simulink model "B2_comparison_tool"  (R2021b)
settings: Solver=VariableStepAuto  StartTime=0.0  StopTime=10  RelTol=1e-3
values from neighbouring files (symbols this model uses):
  K_act = 50    [A10_simple_plant.m]    (also in A11_setup_script_pprz.m = 20; A1_setup_script.m = 20)
  K_act_inner = K_act*eye(4)    [A11_setup_script_pprz.m]    (also in A1_setup_script.m)
  K_ec_u = 1.5    [A11_setup_script_pprz.m]    (also in A1_setup_script.m = 5)
  K_ec_v = 1.5    [A11_setup_script_pprz.m]    (also in A1_setup_script.m = 5)
  K_ec_w = 1.5    [A11_setup_script_pprz.m]    (also in A1_setup_script.m = 5)
  K_u_d = 2.5    [A11_setup_script_pprz.m]    (also in A1_setup_script.m = 7)
  K_v_d = 2.5    [A11_setup_script_pprz.m]    (also in A1_setup_script.m = 7)
  K_w_d = 2.5    [A11_setup_script_pprz.m]    (also in A1_setup_script.m = 7)
  max_motor_rate = 30000    [A11_setup_script_pprz.m]    (also in A1_setup_script.m)
  max_omega_motor = 11000    [A11_setup_script_pprz.m]    (also in A1_setup_script.m)
  omega_c_motors = 50    [A11_setup_script_pprz.m]    (also in A1_setup_script.m)
  sampling_time = 1/frequency    (= 0.002)    [A11_setup_script_pprz.m]    (also in A12_sim_multi_run.m; A1_setup_script.m; A6_slow_actuator.m)
undefined symbols (not defined in the file or in its folder): K_ec_d_p, K_ec_d_q, K_ec_d_r, K_ec_dd_p, K_ec_dd_q, K_ec_dd_r, K_ec_p, K_ec_q, K_ec_r, K_p, K_p_d, K_p_dd, K_q, K_q_d, K_q_dd, K_r, K_r_d, K_r_dd
libraries: dspinverses x16, simulink_extras x8, aerolibutil x2, sharedutil x2, aerolibbdyn x2, aerolibatmos2 x2
(part 4 of 5)

== system B2_comparison_tool/System 1 - Old/INDI w// RSPI/ERROR CONTROLLER VELOCITY ==
  u_ref : Inport
  v_ref : Inport  Port=2
  w_ref : Inport  Port=3
  Gain : Gain  Gain=10
  Gain2 : Gain  Gain=10
  Gain4 : Gain  Gain=10
  Sum : Sum  Inputs=|+-
  Sum3 : Sum  Inputs=|+-
  Sum6 : Sum  Inputs=|+-
  ud_ec : Outport
  vd_ec : Outport  Port=2
  wd_ec : Outport  Port=3
  wires:
  u_ref/1 -> Sum/1
  Sum/1 -> Gain/1
  Gain/1 -> ud_ec/1
  Sum3/1 -> Gain2/1
  v_ref/1 -> Sum3/1
  Gain2/1 -> vd_ec/1
  Sum6/1 -> Gain4/1
  w_ref/1 -> Sum6/1
  [Vx_earth] -> Sum/2
  [Vz_earth] -> Sum6/2
  [Vy_earth] -> Sum3/2
  Gain4/1 -> wd_ec/1

== system B2_comparison_tool/System 1 - Old/INDI w// RSPI/INTERNAL REFERENCE MODEL ATTITUDE ==
  phi_cmd : Inport
  theta_cmd : Inport  Port=2
  psi_cmd : Inport  Port=3
  Gain1 : Gain  Gain=10
  Gain10 : Gain  Gain=20
  Gain11 : Gain  Gain=20
  Gain7 : Gain  Gain=5
  Gain8 : Gain  Gain=20
  Gain9 : Gain  Gain=5
  Integrator{,1..5} (6 alike) : Integrator
  Subsystem : Subsystem
  Subsystem1 : Subsystem
  Sum{1,11,16,20..22} (6 alike) : Sum  Inputs=|+-
  pd_ref : Outport
  qd_ref : Outport  Port=2
  rd_ref : Outport  Port=3
  p_ref : Outport  Port=4
  q_ref : Outport  Port=5
  r_ref : Outport  Port=6
  phi_ref : Outport  Port=7
  theta_ref : Outport  Port=8
  psi_ref : Outport  Port=9
  wires:
  Integrator1/1 -> Sum11/2, theta_ref/1
  Integrator2/1 -> p_ref/1, Subsystem1/1(p), Sum21/2
  Gain11/1 -> rd_ref/1, Integrator4/1
  Subsystem1/1(dphi) -> Integrator3/1
  Subsystem1/3(dpsi) -> Integrator5/1
  Subsystem1/2(dtheta) -> Integrator1/1
  Subsystem/2(q) -> Sum16/1
  Subsystem/1(p) -> Sum21/1
  Gain9/1 -> Subsystem/1(dphi)
  Subsystem/3(r) -> Sum22/1
  Gain8/1 -> qd_ref/1, Integrator/1
  Sum21/1 -> Gain10/1
  Gain7/1 -> Subsystem/2(dtheta)
  Sum11/1 -> Gain7/1
  Sum22/1 -> Gain11/1
  Sum16/1 -> Gain8/1
  Integrator3/1 -> phi_ref/1, Sum20/2
  Sum20/1 -> Gain9/1
  Integrator4/1 -> r_ref/1, Subsystem1/3(r), Sum22/2
  Gain10/1 -> pd_ref/1, Integrator2/1
  Integrator/1 -> q_ref/1, Subsystem1/2(q), Sum16/2
  phi_cmd/1 -> Sum20/1
  theta_cmd/1 -> Sum11/1
  psi_cmd/1 -> Sum1/1
  Integrator5/1 -> Sum1/2, psi_ref/1
  Gain1/1 -> Subsystem/3(dpsi)
  Sum1/1 -> Gain1/1

== system B2_comparison_tool/System 1 - Old/INDI w// RSPI/INTERNAL REFERENCE MODEL VELOCITY ==
  u_cmd : Inport
  v_cmd : Inport  Port=2
  w_cmd : Inport  Port=3
  Gain1 : Gain  Gain=2
  Gain7 : Gain  Gain=2
  Gain9 : Gain  Gain=2
  Integrator1 : Integrator
  Integrator3 : Integrator
  Integrator5 : Integrator
  Sum1 : Sum  Inputs=|+-
  Sum11 : Sum  Inputs=|+-
  Sum20 : Sum  Inputs=|+-
  ud_ref : Outport
  vd_ref : Outport  Port=2
  wd_ref : Outport  Port=3
  u_ref : Outport  Port=4
  v_ref : Outport  Port=5
  w_ref : Outport  Port=6
  wires:
  Integrator1/1 -> w_ref/1, Sum11/2
  Gain7/1 -> Integrator1/1, wd_ref/1
  Gain9/1 -> ud_ref/1, Integrator3/1
  v_cmd/1 -> Sum1/1
  Sum11/1 -> Gain7/1
  Integrator3/1 -> Sum20/2, u_ref/1
  Sum20/1 -> Gain9/1
  u_cmd/1 -> Sum20/1
  w_cmd/1 -> Sum11/1
  Integrator5/1 -> Sum1/2, v_ref/1
  Gain1/1 -> vd_ref/1, Integrator5/1
  Sum1/1 -> Gain1/1

== system B2_comparison_tool/System 0 - New/Equations of Motion/Vehicle Dynamics/Disturbance Block ==
  Step : Step  Time=2  After=60  SampleTime=0
  Sum : Sum  Inputs=|++
  Total Disturbance : Outport
  wires:
  Step/1 -> Sum/1
  Sum/1 -> Total Disturbance/1

== system B2_comparison_tool/System 0 - New/Equations of Motion/Vehicle Dynamics/Omega_I_Omega ==
  pqr_body : Inport
  Inertia : Inport  Port=2
  3x3 Cross Product : sharedutil/3x3 Cross Product  aMode=aMode
      settings: SourceProductBaseCode=AE,PW,DR,MT,UV,VE
  Matrix Multiply1 : Product  Multiplication=Matrix(*)
  Final product : Outport
  wires:
  Inertia/1 -> Matrix Multiply1/1
  Matrix Multiply1/1 -> 3x3 Cross Product/2
  3x3 Cross Product/1 -> Final product/1
  pqr_body/1 -> 3x3 Cross Product/1, Matrix Multiply1/2

== system B2_comparison_tool/System 0 - New/INDI Cascaded/INTERNAL REFERENCE MODEL ATTITUDE/Subsystem ==
  dphi : Inport
  dtheta : Inport  Port=2
  dpsi : Inport  Port=3
  Demux4 : Demux  Outputs=3
  Matrix Multiply2 : Product  Multiplication=Matrix(*)
  Vector Concatenate1 : Concatenate  NumInputs=3
  p : Outport
  q : Outport  Port=2
  r : Outport  Port=3
  wires:
  Vector Concatenate1/1 -> Matrix Multiply2/2
  [R] -> Matrix Multiply2/1
  dphi/1 -> Vector Concatenate1/1
  dtheta/1 -> Vector Concatenate1/2
  Matrix Multiply2/1 -> Demux4/1
  dpsi/1 -> Vector Concatenate1/3
  Demux4/3 -> r/1
  Demux4/1 -> p/1
  Demux4/2 -> q/1

== system B2_comparison_tool/System 0 - New/INDI Cascaded/INTERNAL REFERENCE MODEL ATTITUDE/Subsystem1 ==
  p : Inport
  q : Inport  Port=2
  r : Inport  Port=3
  Demux4 : Demux  Outputs=3
  Matrix Multiply2 : Product  Multiplication=Matrix(*)
  Vector Concatenate1 : Concatenate  NumInputs=3
  dphi : Outport
  dtheta : Outport  Port=2
  dpsi : Outport  Port=3
  wires:
  Vector Concatenate1/1 -> Matrix Multiply2/2
  [R_inv] -> Matrix Multiply2/1
  p/1 -> Vector Concatenate1/1
  q/1 -> Vector Concatenate1/2
  Matrix Multiply2/1 -> Demux4/1
  r/1 -> Vector Concatenate1/3
  Demux4/3 -> dpsi/1
  Demux4/1 -> dphi/1
  Demux4/2 -> dtheta/1

== system B2_comparison_tool/System 0 - New/INDI Cascaded w// Actuator Consideration/INTERNAL REFERENCE MODEL ATTITUDE/Subsystem ==
  dphi : Inport
  dtheta : Inport  Port=2
  dpsi : Inport  Port=3
  Demux4 : Demux  Outputs=3
  Matrix Multiply2 : Product  Multiplication=Matrix(*)
  Vector Concatenate1 : Concatenate  NumInputs=3
  p : Outport
  q : Outport  Port=2
  r : Outport  Port=3
  wires:
  Vector Concatenate1/1 -> Matrix Multiply2/2
  [R] -> Matrix Multiply2/1
  dphi/1 -> Vector Concatenate1/1
  dtheta/1 -> Vector Concatenate1/2
  Matrix Multiply2/1 -> Demux4/1
  dpsi/1 -> Vector Concatenate1/3
  Demux4/3 -> r/1
  Demux4/1 -> p/1
  Demux4/2 -> q/1

== system B2_comparison_tool/System 0 - New/INDI Cascaded w// Actuator Consideration/INTERNAL REFERENCE MODEL ATTITUDE/Subsystem1 ==
  p : Inport
  q : Inport  Port=2
  r : Inport  Port=3
  Demux4 : Demux  Outputs=3
  Matrix Multiply2 : Product  Multiplication=Matrix(*)
  Vector Concatenate1 : Concatenate  NumInputs=3
  dphi : Outport
  dtheta : Outport  Port=2
  dpsi : Outport  Port=3
  wires:
  Vector Concatenate1/1 -> Matrix Multiply2/2
  [R_inv] -> Matrix Multiply2/1
  p/1 -> Vector Concatenate1/1
  q/1 -> Vector Concatenate1/2
  Matrix Multiply2/1 -> Demux4/1
  r/1 -> Vector Concatenate1/3
  Demux4/3 -> dpsi/1
  Demux4/1 -> dphi/1
  Demux4/2 -> dtheta/1

== system B2_comparison_tool/System 0 - New/INDI Cascaded w// State Compensation on qdd/INTERNAL REFERENCE MODEL ATTITUDE/Subsystem ==
  dphi : Inport
  dtheta : Inport  Port=2
  dpsi : Inport  Port=3
  Demux4 : Demux  Outputs=3
  Matrix Multiply2 : Product  Multiplication=Matrix(*)
  Vector Concatenate1 : Concatenate  NumInputs=3
  p : Outport
  q : Outport  Port=2
  r : Outport  Port=3
  wires:
  Vector Concatenate1/1 -> Matrix Multiply2/2
  [R] -> Matrix Multiply2/1
  dphi/1 -> Vector Concatenate1/1
  dtheta/1 -> Vector Concatenate1/2
  Matrix Multiply2/1 -> Demux4/1
  dpsi/1 -> Vector Concatenate1/3
  Demux4/3 -> r/1
  Demux4/1 -> p/1
  Demux4/2 -> q/1

== system B2_comparison_tool/System 0 - New/INDI Cascaded w// State Compensation on qdd/INTERNAL REFERENCE MODEL ATTITUDE/Subsystem1 ==
  p : Inport
  q : Inport  Port=2
  r : Inport  Port=3
  Demux4 : Demux  Outputs=3
  Matrix Multiply2 : Product  Multiplication=Matrix(*)
  Vector Concatenate1 : Concatenate  NumInputs=3
  dphi : Outport
  dtheta : Outport  Port=2
  dpsi : Outport  Port=3
  wires:
  Vector Concatenate1/1 -> Matrix Multiply2/2
  [R_inv] -> Matrix Multiply2/1
  p/1 -> Vector Concatenate1/1
  q/1 -> Vector Concatenate1/2
  Matrix Multiply2/1 -> Demux4/1
  r/1 -> Vector Concatenate1/3
  Demux4/3 -> dpsi/1
  Demux4/1 -> dphi/1
  Demux4/2 -> dtheta/1

== system B2_comparison_tool/System 0 - New/INDI Cascaded w// State Compensation on qdd/STATE COMPENSATION BLOCK/Moment Block form Plant - Plant States ==
  Aerodynamic Forces Calculator : MATLAB Function  TreatAsAtomicUnit=on
  Divide : Product  Inputs=*/
  Radians to Degrees : simulink_extras/Transformations/Radians to Degrees
  Radians to Degrees1 : simulink_extras/Transformations/Radians to Degrees
  Scope1 : Scope  NumInputPorts=2
  Scope2 : Scope  NumInputPorts=2
  Scope3 : Scope  NumInputPorts=2
  Terminator{,1..3,5} (5 alike) : Terminator
  qd : Outport
  wires:
  Radians to Degrees1/1 -> Scope3/2
  Aerodynamic Forces Calculator/11(alpha) -> Radians to Degrees/1  "alpha"
  [rho] -> Aerodynamic Forces Calculator/4(rho)
  Aerodynamic Forces Calculator/8(Cd) -> Scope1/2  "Cd"
  [r_plate] -> Aerodynamic Forces Calculator/5(r_plate)
  Aerodynamic Forces Calculator/9(L) -> Scope2/1  "L"
  [Vz_body] -> Aerodynamic Forces Calculator/3(zd_body)
  Aerodynamic Forces Calculator/7(Cl) -> Scope1/1  "Cl"
  Aerodynamic Forces Calculator/10(D) -> Scope2/2  "D"
  Aerodynamic Forces Calculator/12(beta) -> Radians to Degrees1/1  "beta"
  [l_plate] -> Aerodynamic Forces Calculator/6(l_plate)
  [Vx_body] -> Aerodynamic Forces Calculator/1(xd_body)
  [Vy_body] -> Aerodynamic Forces Calculator/2(yd_body)
  Radians to Degrees/1 -> Scope3/1
  Aerodynamic Forces Calculator/1(Fx_body) -> Terminator/1  "Fx_body"
  Aerodynamic Forces Calculator/2(Fy_body) -> Terminator1/1  "Fy_body"
  Aerodynamic Forces Calculator/3(Fz_body) -> Terminator2/1  "Fz_body"
  Aerodynamic Forces Calculator/4(L_aero) -> Terminator3/1  "Mx"
  Aerodynamic Forces Calculator/5(M_aero) -> Divide/1  "My"
  Aerodynamic Forces Calculator/6(N_aero) -> Terminator5/1  "Mz"
  [Iyy] -> Divide/2
  Divide/1 -> qd/1

== system B2_comparison_tool/System 0 - New/INDI Cascaded w// State Compensation on qdd/STATE COMPENSATION BLOCK/Moment Block form Plant - Reference States  ==
  Aerodynamic Forces Calculator : MATLAB Function  TreatAsAtomicUnit=on
  Demux : Demux  Outputs=3
  Divide : Product  Inputs=*/
  MatrixMultiply : Product  Multiplication=Matrix(*)
  Mux : Mux  Inputs=3
  Radians to Degrees : simulink_extras/Transformations/Radians to Degrees
  Radians to Degrees1 : simulink_extras/Transformations/Radians to Degrees
  Scope1 : Scope  NumInputPorts=2
  Scope2 : Scope  NumInputPorts=2
  Scope3 : Scope  NumInputPorts=2
  Terminator{,1..3,5} (5 alike) : Terminator
  Transpose : Math  Operator=transpose  SaturateOnIntegerOverflow=on
  qd : Outport
  wires:
  Radians to Degrees1/1 -> Scope3/2
  Aerodynamic Forces Calculator/11(alpha) -> Radians to Degrees/1  "alpha"
  [rho] -> Aerodynamic Forces Calculator/4(rho)
  Aerodynamic Forces Calculator/8(Cd) -> Scope1/2  "Cd"
  [r_plate] -> Aerodynamic Forces Calculator/5(r_plate)
  Aerodynamic Forces Calculator/9(L) -> Scope2/1  "L"
  Aerodynamic Forces Calculator/7(Cl) -> Scope1/1  "Cl"
  Aerodynamic Forces Calculator/10(D) -> Scope2/2  "D"
  Aerodynamic Forces Calculator/12(beta) -> Radians to Degrees1/1  "beta"
  [l_plate] -> Aerodynamic Forces Calculator/6(l_plate)
  Radians to Degrees/1 -> Scope3/1
  Aerodynamic Forces Calculator/1(Fx_body) -> Terminator/1  "Fx_body"
  Aerodynamic Forces Calculator/2(Fy_body) -> Terminator1/1  "Fy_body"
  Aerodynamic Forces Calculator/3(Fz_body) -> Terminator2/1  "Fz_body"
  Aerodynamic Forces Calculator/4(L_aero) -> Terminator3/1  "Mx"
  Aerodynamic Forces Calculator/5(M_aero) -> Divide/1  "My"
  Aerodynamic Forces Calculator/6(N_aero) -> Terminator5/1  "Mz"
  [Iyy] -> Divide/2
  Divide/1 -> qd/1
  [R_bg] -> Transpose/1
  Transpose/1 -> MatrixMultiply/1
  [Vy_earth_ref] -> Mux/2
  [Vx_earth_ref] -> Mux/1
  [Vz_earth_ref] -> Mux/3
  Mux/1 -> MatrixMultiply/2
  MatrixMultiply/1 -> Demux/1
  Demux/2 -> Aerodynamic Forces Calculator/2(yd_body)
  Demux/1 -> Aerodynamic Forces Calculator/1(xd_body)
  Demux/3 -> Aerodynamic Forces Calculator/3(zd_body)

== system B2_comparison_tool/System 0 - New/INDI w// RSPI/INTERNAL REFERENCE MODEL ATTITUDE/Subsystem ==
  dphi : Inport
  dtheta : Inport  Port=2
  dpsi : Inport  Port=3
  Demux4 : Demux  Outputs=3
  Matrix Multiply2 : Product  Multiplication=Matrix(*)
  Vector Concatenate1 : Concatenate  NumInputs=3
  p : Outport
  q : Outport  Port=2
  r : Outport  Port=3
  wires:
  Vector Concatenate1/1 -> Matrix Multiply2/2
  [R] -> Matrix Multiply2/1
  dphi/1 -> Vector Concatenate1/1
  dtheta/1 -> Vector Concatenate1/2
  Matrix Multiply2/1 -> Demux4/1
  dpsi/1 -> Vector Concatenate1/3
  Demux4/3 -> r/1
  Demux4/1 -> p/1
  Demux4/2 -> q/1

== system B2_comparison_tool/System 0 - New/INDI w// RSPI/INTERNAL REFERENCE MODEL ATTITUDE/Subsystem1 ==
  p : Inport
  q : Inport  Port=2
  r : Inport  Port=3
  Demux4 : Demux  Outputs=3
  Matrix Multiply2 : Product  Multiplication=Matrix(*)
  Vector Concatenate1 : Concatenate  NumInputs=3
  dphi : Outport
  dtheta : Outport  Port=2
  dpsi : Outport  Port=3
  wires:
  Vector Concatenate1/1 -> Matrix Multiply2/2
  [R_inv] -> Matrix Multiply2/1
  p/1 -> Vector Concatenate1/1
  q/1 -> Vector Concatenate1/2
  Matrix Multiply2/1 -> Demux4/1
  r/1 -> Vector Concatenate1/3
  Demux4/3 -> dpsi/1
  Demux4/1 -> dphi/1
  Demux4/2 -> dtheta/1

== system B2_comparison_tool/System 1 - Old/Equations of Motion/Vehicle Dynamics/Disturbance Block ==
  Step : Step  Time=2  After=60  SampleTime=0
  Step1 : Step  Time=6  After=8  SampleTime=0
  Sum : Sum  Inputs=|++
  Total Disturbance : Outport
  wires:
  Step/1 -> Sum/1
  Sum/1 -> Total Disturbance/1
  Step1/1 -> ?

== system B2_comparison_tool/System 1 - Old/Equations of Motion/Vehicle Dynamics/Omega_I_Omega ==
  pqr_body : Inport
  Inertia : Inport  Port=2
  3x3 Cross Product : sharedutil/3x3 Cross Product  aMode=aMode
      settings: SourceProductBaseCode=AE,PW,DR,MT,UV,VE
  Matrix Multiply1 : Product  Multiplication=Matrix(*)
  Final product : Outport
  wires:
  Inertia/1 -> Matrix Multiply1/1
  Matrix Multiply1/1 -> 3x3 Cross Product/2
  3x3 Cross Product/1 -> Final product/1
  pqr_body/1 -> 3x3 Cross Product/1, Matrix Multiply1/2

== system B2_comparison_tool/System 1 - Old/INDI Cascaded/INTERNAL REFERENCE MODEL ATTITUDE/Subsystem ==
  dphi : Inport
  dtheta : Inport  Port=2
  dpsi : Inport  Port=3
  Demux4 : Demux  Outputs=3
  Matrix Multiply2 : Product  Multiplication=Matrix(*)
  Vector Concatenate1 : Concatenate  NumInputs=3
  p : Outport
  q : Outport  Port=2
  r : Outport  Port=3
  wires:
  Vector Concatenate1/1 -> Matrix Multiply2/2
  [R] -> Matrix Multiply2/1
  dphi/1 -> Vector Concatenate1/1
  dtheta/1 -> Vector Concatenate1/2
  Matrix Multiply2/1 -> Demux4/1
  dpsi/1 -> Vector Concatenate1/3
  Demux4/3 -> r/1
  Demux4/1 -> p/1
  Demux4/2 -> q/1

== system B2_comparison_tool/System 1 - Old/INDI Cascaded/INTERNAL REFERENCE MODEL ATTITUDE/Subsystem1 ==
  p : Inport
  q : Inport  Port=2
  r : Inport  Port=3
  Demux4 : Demux  Outputs=3
  Matrix Multiply2 : Product  Multiplication=Matrix(*)
  Vector Concatenate1 : Concatenate  NumInputs=3
  dphi : Outport
  dtheta : Outport  Port=2
  dpsi : Outport  Port=3
  wires:
  Vector Concatenate1/1 -> Matrix Multiply2/2
  [R_inv] -> Matrix Multiply2/1
  p/1 -> Vector Concatenate1/1
  q/1 -> Vector Concatenate1/2
  Matrix Multiply2/1 -> Demux4/1
  r/1 -> Vector Concatenate1/3
  Demux4/3 -> dpsi/1
  Demux4/1 -> dphi/1
  Demux4/2 -> dtheta/1

== system B2_comparison_tool/System 1 - Old/INDI Cascaded w// Actuator Consideration/INTERNAL REFERENCE MODEL ATTITUDE/Subsystem ==
  dphi : Inport
  dtheta : Inport  Port=2
  dpsi : Inport  Port=3
  Demux4 : Demux  Outputs=3
  Matrix Multiply2 : Product  Multiplication=Matrix(*)
  Vector Concatenate1 : Concatenate  NumInputs=3
  p : Outport
  q : Outport  Port=2
  r : Outport  Port=3
  wires:
  Vector Concatenate1/1 -> Matrix Multiply2/2
  [R] -> Matrix Multiply2/1
  dphi/1 -> Vector Concatenate1/1
  dtheta/1 -> Vector Concatenate1/2
  Matrix Multiply2/1 -> Demux4/1
  dpsi/1 -> Vector Concatenate1/3
  Demux4/3 -> r/1
  Demux4/1 -> p/1
  Demux4/2 -> q/1

== system B2_comparison_tool/System 1 - Old/INDI Cascaded w// Actuator Consideration/INTERNAL REFERENCE MODEL ATTITUDE/Subsystem1 ==
  p : Inport
  q : Inport  Port=2
  r : Inport  Port=3
  Demux4 : Demux  Outputs=3
  Matrix Multiply2 : Product  Multiplication=Matrix(*)
  Vector Concatenate1 : Concatenate  NumInputs=3
  dphi : Outport
  dtheta : Outport  Port=2
  dpsi : Outport  Port=3
  wires:
  Vector Concatenate1/1 -> Matrix Multiply2/2
  [R_inv] -> Matrix Multiply2/1
  p/1 -> Vector Concatenate1/1
  q/1 -> Vector Concatenate1/2
  Matrix Multiply2/1 -> Demux4/1
  r/1 -> Vector Concatenate1/3
  Demux4/3 -> dpsi/1
  Demux4/1 -> dphi/1
  Demux4/2 -> dtheta/1

== system B2_comparison_tool/System 1 - Old/INDI w// RSPI/INTERNAL REFERENCE MODEL ATTITUDE/Subsystem ==
  dphi : Inport
  dtheta : Inport  Port=2
  dpsi : Inport  Port=3
  Demux4 : Demux  Outputs=3
  Matrix Multiply2 : Product  Multiplication=Matrix(*)
  Vector Concatenate1 : Concatenate  NumInputs=3
  p : Outport
  q : Outport  Port=2
  r : Outport  Port=3
  wires:
  Vector Concatenate1/1 -> Matrix Multiply2/2
  [R] -> Matrix Multiply2/1
  dphi/1 -> Vector Concatenate1/1
  dtheta/1 -> Vector Concatenate1/2
  Matrix Multiply2/1 -> Demux4/1
  dpsi/1 -> Vector Concatenate1/3
  Demux4/3 -> r/1
  Demux4/1 -> p/1
  Demux4/2 -> q/1

== system B2_comparison_tool/System 1 - Old/INDI w// RSPI/INTERNAL REFERENCE MODEL ATTITUDE/Subsystem1 ==
  p : Inport
  q : Inport  Port=2
  r : Inport  Port=3
  Demux4 : Demux  Outputs=3
  Matrix Multiply2 : Product  Multiplication=Matrix(*)
  Vector Concatenate1 : Concatenate  NumInputs=3
  dphi : Outport
  dtheta : Outport  Port=2
  dpsi : Outport  Port=3
  wires:
  Vector Concatenate1/1 -> Matrix Multiply2/2
  [R_inv] -> Matrix Multiply2/1
  p/1 -> Vector Concatenate1/1
  q/1 -> Vector Concatenate1/2
  Matrix Multiply2/1 -> Demux4/1
  r/1 -> Vector Concatenate1/3
  Demux4/3 -> dpsi/1
  Demux4/1 -> dphi/1
  Demux4/2 -> dtheta/1

== matlab function B2_comparison_tool/System 0 - New/INDI Cascaded w// State Compensation on qdd/MATLAB Function ==
  data: Ixx input; B_inner output; Iyy input; Izz input; K_m input; K_t input; Omega_1 input; Omega_2 input; Omega_3 input; Omega_4 input; b input; l input; K_act_inner input
function B_inner = control_allocation_simple_inner(Ixx,Iyy,Izz,K_m,K_t,Omega_1,Omega_2,Omega_3,Omega_4,b,l,K_act_inner)

B_inner = zeros(4,4);

B_inner(1,1) = -(2*K_t*Omega_1*b)/Ixx;
B_inner(1,2) = (2*K_t*Omega_2*b)/Ixx;
B_inner(1,3) = (2*K_t*Omega_3*b)/Ixx;
B_inner(1,4) = -(2*K_t*Omega_4*b)/Ixx;

B_inner(2,1) = (2*K_t*Omega_1*l)/Iyy;
B_inner(2,2) = (2*K_t*Omega_2*l)/Iyy;
B_inner(2,3) = -(2*K_t*Omega_3*l)/Iyy;
B_inner(2,4) = -(2*K_t*Omega_4*l)/Iyy;

B_inner(3,1) = (2*K_m*Omega_1)/Izz;
B_inner(3,2) = -(2*K_m*Omega_2)/Izz;
B_inner(3,3) = (2*K_m*Omega_3)/Izz;
B_inner(3,4) = -(2*K_m*Omega_4)/Izz;

B_inner(4,1) = -2*K_t*Omega_1;
B_inner(4,2) = -2*K_t*Omega_2;
B_inner(4,3) = -2*K_t*Omega_3;
B_inner(4,4) = -2*K_t*Omega_4;

% actuator compensation
B_inner = K_act_inner*B_inner;

end

== matlab function B2_comparison_tool/System 0 - New/Equations of Motion/Vehicle Dynamics/pqr_to_euler_rates ==
  data: Phi input; T output; Theta input
function T = pqr_to_euler_rates(Phi,Theta)
y=[ 1  sin(Phi)*tan(Theta)  cos(Phi)*tan(Theta)  ;
    0       cos(Phi)             -sin(Phi)       ;
    0  sin(Phi)*sec(Theta)   cos(Phi)*sec(Theta)];
T = y;

== matlab function B2_comparison_tool/System 0 - New/INDI Cascaded w// Actuator Consideration/MATLAB Function ==
  data: Ixx input; B_inner output; Iyy input; Izz input; K_m input; K_t input; Omega_1 input; Omega_2 input; Omega_3 input; Omega_4 input; b input; l input; K_act_inner input
function B_inner = control_allocation_simple_inner(Ixx,Iyy,Izz,K_m,K_t,Omega_1,Omega_2,Omega_3,Omega_4,b,l,K_act_inner)

B_inner = zeros(4,4);

B_inner(1,1) = -(2*K_t*Omega_1*b)/Ixx;
B_inner(1,2) = (2*K_t*Omega_2*b)/Ixx;
B_inner(1,3) = (2*K_t*Omega_3*b)/Ixx;
B_inner(1,4) = -(2*K_t*Omega_4*b)/Ixx;

B_inner(2,1) = (2*K_t*Omega_1*l)/Iyy;
B_inner(2,2) = (2*K_t*Omega_2*l)/Iyy;
B_inner(2,3) = -(2*K_t*Omega_3*l)/Iyy;
B_inner(2,4) = -(2*K_t*Omega_4*l)/Iyy;

B_inner(3,1) = (2*K_m*Omega_1)/Izz;
B_inner(3,2) = -(2*K_m*Omega_2)/Izz;
B_inner(3,3) = (2*K_m*Omega_3)/Izz;
B_inner(3,4) = -(2*K_m*Omega_4)/Izz;

B_inner(4,1) = -2*K_t*Omega_1;
B_inner(4,2) = -2*K_t*Omega_2;
B_inner(4,3) = -2*K_t*Omega_3;
B_inner(4,4) = -2*K_t*Omega_4;

% actuator compensation
B_inner = K_act_inner*B_inner;

end

== matlab function B2_comparison_tool/System 0 - New/Equations of Motion/Vehicle Dynamics/body_to_ground_transorm ==
  data: Phi input; R_bg output; Theta input; Psi input
function R_bg  = R_bg(Phi,Theta,Psi)
y = [cos(Theta)*cos(Psi)   -cos(Phi)*sin(Psi)+sin(Phi)*sin(Theta)*cos(Psi)  sin(Phi)*sin(Psi)+cos(Phi)*sin(Theta)*cos(Psi) ;
     +cos(Theta)*sin(Psi)  cos(Phi)*cos(Psi)+sin(Phi)*sin(Theta)*sin(Psi)  -sin(Phi)*cos(Psi)+cos(Phi)*sin(Theta)*sin(Psi) ;
       -sin(Theta)                        +sin(Phi)*cos(Theta)              cos(Phi)*cos(Theta)                             ];
R_bg = y;

== matlab function B2_comparison_tool/System 0 - New/INDI Cascaded w// Actuator Consideration/MATLAB Function1 ==
  data: T input; B_outer output; Phi input; Theta input; Psi input; m input
function B_outer = control_allocation_simple_outer(T,Phi,Theta,Psi,m)

B_outer = zeros(3,3);

B_outer(1,1) = (T*(cos(Phi)*sin(Psi) - cos(Psi)*sin(Phi)*sin(Theta)))/m;  
B_outer(1,2) = (T*cos(Phi)*cos(Psi)*cos(Theta))/m;
B_outer(1,3) = (sin(Phi)*sin(Psi) + cos(Phi)*cos(Psi)*sin(Theta))/m;

B_outer(2,1) = -(T*(cos(Phi)*cos(Psi) + sin(Phi)*sin(Psi)*sin(Theta)))/m;
B_outer(2,2) = (T*cos(Phi)*cos(Theta)*sin(Psi))/m;
B_outer(2,3) = -(cos(Psi)*sin(Phi) - cos(Phi)*sin(Psi)*sin(Theta))/m;

B_outer(3,1) = -(T*cos(Theta)*sin(Phi))/m;                         
B_outer(3,2) = -(T*cos(Phi)*sin(Theta))/m;
B_outer(3,3) = (cos(Phi)*cos(Theta))/m; 

end

== matlab function B2_comparison_tool/System 0 - New/INDI Cascaded w// PD controller/MATLAB Function ==
  data: Ixx input; B_inner output; Iyy input; Izz input; K_m input; K_t input; Omega_1 input; Omega_2 input; Omega_3 input; Omega_4 input; b input; l input
function B_inner = control_allocation_simple_inner(Ixx,Iyy,Izz,K_m,K_t,Omega_1,Omega_2,Omega_3,Omega_4,b,l)

B_inner = zeros(4,4);

B_inner(1,1) = -(2*K_t*Omega_1*b)/Ixx;
B_inner(1,2) = (2*K_t*Omega_2*b)/Ixx;
B_inner(1,3) = (2*K_t*Omega_3*b)/Ixx;
B_inner(1,4) = -(2*K_t*Omega_4*b)/Ixx;

B_inner(2,1) = (2*K_t*Omega_1*l)/Iyy;
B_inner(2,2) = (2*K_t*Omega_2*l)/Iyy;
B_inner(2,3) = -(2*K_t*Omega_3*l)/Iyy;
B_inner(2,4) = -(2*K_t*Omega_4*l)/Iyy;

B_inner(3,1) = (2*K_m*Omega_1)/Izz;
B_inner(3,2) = -(2*K_m*Omega_2)/Izz;
B_inner(3,3) = (2*K_m*Omega_3)/Izz;
B_inner(3,4) = -(2*K_m*Omega_4)/Izz;

B_inner(4,1) = -2*K_t*Omega_1;
B_inner(4,2) = -2*K_t*Omega_2;
B_inner(4,3) = -2*K_t*Omega_3;
B_inner(4,4) = -2*K_t*Omega_4;

end

== matlab function B2_comparison_tool/System 0 - New/INDI Cascaded w// PD controller/MATLAB Function1 ==
  data: T input; B_outer output; Phi input; Theta input; Psi input; m input
function B_outer = control_allocation_simple_outer(T,Phi,Theta,Psi,m)

B_outer = zeros(3,3);

B_outer(1,1) = (T*(cos(Phi)*sin(Psi) - cos(Psi)*sin(Phi)*sin(Theta)))/m;  
B_outer(1,2) = (T*cos(Phi)*cos(Psi)*cos(Theta))/m;
B_outer(1,3) = (sin(Phi)*sin(Psi) + cos(Phi)*cos(Psi)*sin(Theta))/m;

B_outer(2,1) = -(T*(cos(Phi)*cos(Psi) + sin(Phi)*sin(Psi)*sin(Theta)))/m;
B_outer(2,2) = (T*cos(Phi)*cos(Theta)*sin(Psi))/m;
B_outer(2,3) = -(cos(Psi)*sin(Phi) - cos(Phi)*sin(Psi)*sin(Theta))/m;

B_outer(3,1) = -(T*cos(Theta)*sin(Phi))/m;                         
B_outer(3,2) = -(T*cos(Phi)*sin(Theta))/m;
B_outer(3,3) = (cos(Phi)*cos(Theta))/m; 

end

== matlab function B2_comparison_tool/System 0 - New/INDI Cascaded/MATLAB Function ==
  data: Ixx input; B_inner output; Iyy input; Izz input; K_m input; K_t input; Omega_1 input; Omega_2 input; Omega_3 input; Omega_4 input; b input; l input
function B_inner = control_allocation_simple_inner(Ixx,Iyy,Izz,K_m,K_t,Omega_1,Omega_2,Omega_3,Omega_4,b,l)

B_inner = zeros(4,4);

B_inner(1,1) = -(2*K_t*Omega_1*b)/Ixx;
B_inner(1,2) = (2*K_t*Omega_2*b)/Ixx;
B_inner(1,3) = (2*K_t*Omega_3*b)/Ixx;
B_inner(1,4) = -(2*K_t*Omega_4*b)/Ixx;

B_inner(2,1) = (2*K_t*Omega_1*l)/Iyy;
B_inner(2,2) = (2*K_t*Omega_2*l)/Iyy;
B_inner(2,3) = -(2*K_t*Omega_3*l)/Iyy;
B_inner(2,4) = -(2*K_t*Omega_4*l)/Iyy;

B_inner(3,1) = (2*K_m*Omega_1)/Izz;
B_inner(3,2) = -(2*K_m*Omega_2)/Izz;
B_inner(3,3) = (2*K_m*Omega_3)/Izz;
B_inner(3,4) = -(2*K_m*Omega_4)/Izz;

B_inner(4,1) = -2*K_t*Omega_1;
B_inner(4,2) = -2*K_t*Omega_2;
B_inner(4,3) = -2*K_t*Omega_3;
B_inner(4,4) = -2*K_t*Omega_4;

end

== matlab function B2_comparison_tool/System 0 - New/INDI Cascaded/MATLAB Function1 ==
  data: T input; B_outer output; Phi input; Theta input; Psi input; m input
function B_outer = control_allocation_simple_outer(T,Phi,Theta,Psi,m)

B_outer = zeros(3,3);

B_outer(1,1) = (T*(cos(Phi)*sin(Psi) - cos(Psi)*sin(Phi)*sin(Theta)))/m;  
B_outer(1,2) = (T*cos(Phi)*cos(Psi)*cos(Theta))/m;
B_outer(1,3) = (sin(Phi)*sin(Psi) + cos(Phi)*cos(Psi)*sin(Theta))/m;

B_outer(2,1) = -(T*(cos(Phi)*cos(Psi) + sin(Phi)*sin(Psi)*sin(Theta)))/m;
B_outer(2,2) = (T*cos(Phi)*cos(Theta)*sin(Psi))/m;
B_outer(2,3) = -(cos(Psi)*sin(Phi) - cos(Phi)*sin(Psi)*sin(Theta))/m;

B_outer(3,1) = -(T*cos(Theta)*sin(Phi))/m;                         
B_outer(3,2) = -(T*cos(Phi)*sin(Theta))/m;
B_outer(3,3) = (cos(Phi)*cos(Theta))/m; 

end

== matlab function B2_comparison_tool/System 1 - Old/Equations of Motion/Vehicle Dynamics/body_to_ground_transorm ==
  data: Phi input; R_bg output; Theta input; Psi input
function R_bg  = R_bg(Phi,Theta,Psi)
y = [cos(Theta)*cos(Psi)   -cos(Phi)*sin(Psi)+sin(Phi)*sin(Theta)*cos(Psi)  sin(Phi)*sin(Psi)+cos(Phi)*sin(Theta)*cos(Psi) ;
     +cos(Theta)*sin(Psi)  cos(Phi)*cos(Psi)+sin(Phi)*sin(Theta)*sin(Psi)  -sin(Phi)*cos(Psi)+cos(Phi)*sin(Theta)*sin(Psi) ;
       -sin(Theta)                        +sin(Phi)*cos(Theta)              cos(Phi)*cos(Theta)                             ];
R_bg = y;

== matlab function B2_comparison_tool/System 1 - Old/Equations of Motion/Vehicle Dynamics/euler_rates_to_pqr ==
  data: Phi input; R output; Theta input
function R = euler_rates_to_pqr(Phi,Theta)
y=[ 1 0 -sin(Theta);
    0 cos(Phi) sin(Phi)*cos(Theta);
    0 -sin(Phi) cos(Phi)*cos(Theta)];
R = y;

== matlab function B2_comparison_tool/System 0 - New/Equations of Motion/Vehicle Dynamics/euler_rates_to_pqr ==
  data: Phi input; R output; Theta input
function R = euler_rates_to_pqr(Phi,Theta)
y=[ 1 0 -sin(Theta);
    0 cos(Phi) sin(Phi)*cos(Theta);
    0 -sin(Phi) cos(Phi)*cos(Theta)];
R = y;

== matlab function B2_comparison_tool/System 1 - Old/Equations of Motion/Vehicle Dynamics/pqr_to_euler_rates ==
  data: Phi input; T output; Theta input
function T = pqr_to_euler_rates(Phi,Theta)
y=[ 1  sin(Phi)*tan(Theta)  cos(Phi)*tan(Theta)  ;
    0       cos(Phi)             -sin(Phi)       ;
    0  sin(Phi)*sec(Theta)   cos(Phi)*sec(Theta)];
T = y;

== matlab function B2_comparison_tool/System 1 - Old/Force and Moment Calculation/Forces and Moments due to Aerodynamic Forces/Aerodynamic Forces Calculator ==
  data: xd_body input; Fx_body output; yd_body input; zd_body input; Fy_body output; Fz_body output; L_aero output; M_aero output; N_aero output; rho input; r_plate input; l_plate input; Cl output; Cd output; L output; D output; alpha output; beta output
function [Fx_body, Fy_body, Fz_body, L_aero, M_aero, N_aero, Cl, Cd, L, D, alpha, beta] = aero_forces(xd_body,yd_body,zd_body,rho,r_plate,l_plate)
%% Function to estimate the total aerodynamic force acting on the Quad

% initiate values
Fx_body = 0;
Fy_body = 0;
Fz_body = 0;
L_aero = 0;
M_aero = 0;
N_aero = 0;
Cl = 0;
Cd = 0;
L = 0;
D = 0;
beta = 0;

% Find speed vector in path direction
V_t = sqrt(xd_body^2+yd_body^2+zd_body^2);

% Plate area
S_plate = pi*r_plate^2;

% Protection from alpha singularities
if (abs(zd_body) < 0.001 || abs(xd_body) < 0.001)
    alpha = 0;
else
    alpha = atan2(zd_body, xd_body);

% Find the aerodynamics angles between flight path and body orientation

beta = 0;

% Drag Coefficient
Cd = 0.0033*(90+rad2deg(alpha))+0.7;

% Lift Coefficient
Cl = -0.0228*(90+rad2deg(alpha))+2.01;

% Lateral Coefficients
% Cy = 0;

% Calculate actual forces on the body frame
L = 0.5 * rho * V_t^2 * S_plate * Cl;
D = 0.5 * rho * V_t^2 * S_plate * Cd;
% Y = 0.5 * rho * V_t^2 * S_plate * 0;
% Fx_body = (- D * cos(alpha) * cos(beta) + L * sin(alpha) -Y * cos(alpha) * cos(beta))*sign(xd_body);
% Fy_body = Y * cos(beta) - D * sin(beta);
% Fz_body = - L * cos(alpha) - D * sin(alpha) * cos(beta) - Y * sin(alpha) * sin(beta);

Fx_body = (- D*cos(alpha) + L*sin(alpha))*sign(xd_body);
Fy_body = 0;
Fz_body = (L*cos(alpha) - D*sin(alpha));

% Calculate the moment forces acting on the quad
L_aero = 0;
M_aero = l_plate * (D*cos(alpha)-L*sin(alpha));
N_aero = 0;
end

== matlab function B2_comparison_tool/System 1 - Old/Force and Moment Calculation/Forces due to thrust ==
  data: omega_1 input; omega_2 input; F_t_e output; omega_3 input; omega_4 input; R_bg input; K_t input; F_t_b output
function [F_t_e,F_t_b] = F_t(omega_1, omega_2, omega_3, omega_4, R_bg, K_t)

f_1 = [0 0 -K_t * omega_1^2];
f_2 = [0 0 -K_t * omega_2^2]; 
f_3 = [0 0 -K_t * omega_3^2]; 
f_4 = [0 0 -K_t * omega_4^2];

F_t_e = R_bg * (f_1' + f_2' + f_3' + f_4');
F_t_b = (f_1(:,3) + f_2(:,3) + f_3(:,3) + f_4(:,3));

== matlab function B2_comparison_tool/System 1 - Old/Force and Moment Calculation/Moments due to thrust ==
  data: omega_1 input; omega_2 input; M_t output; omega_3 input; omega_4 input; K_t input; K_m input; b input; l input
function M_t = M_t(omega_1, omega_2, omega_3, omega_4, K_t, K_m, b, l)

% forces and torques applied by the propellers in the body frame
t_1 = omega_1^2;
t_2 = omega_2^2;
t_3 = omega_3^2;
t_4 = omega_4^2;
omega_vector = [t_1 t_2 t_3 t_4];

% matrix moments
M_t_matrix = [-b*K_t b*K_t b*K_t -b*K_t;
              l*K_t l*K_t -l*K_t -l*K_t;
              K_m -K_m K_m -K_m];

M_t = M_t_matrix * omega_vector';

== matlab function B2_comparison_tool/System 1 - Old/INDI Block/MATLAB Function ==
  data: Ixx input; B_out output; Iyy input; Izz input; K_m input; K_t input; Omega_1 input; Omega_2 input; Omega_3 input; Omega_4 input; Phi input; Psi input; Theta input; b input; l input; m input
function B_out = control_allocation_simple(Ixx,Iyy,Izz,K_m,K_t,Omega_1,Omega_2,Omega_3,Omega_4,Phi,Psi,Theta,b,l,m)

B_out = zeros(6,4);

B_out(1,1) = -(2*K_t*Omega_1*(sin(Phi)*sin(Psi) + cos(Phi)*cos(Psi)*sin(Theta)))/m;
B_out(1,2) = -(2*K_t*Omega_2*(sin(Phi)*sin(Psi) + cos(Phi)*cos(Psi)*sin(Theta)))/m;
B_out(1,3) = -(2*K_t*Omega_3*(sin(Phi)*sin(Psi) + cos(Phi)*cos(Psi)*sin(Theta)))/m;
B_out(1,4) = -(2*K_t*Omega_4*(sin(Phi)*sin(Psi) + cos(Phi)*cos(Psi)*sin(Theta)))/m;

B_out(2,1) = (2*K_t*Omega_1*(cos(Psi)*sin(Phi) - cos(Phi)*sin(Psi)*sin(Theta)))/m;
B_out(2,2) = (2*K_t*Omega_2*(cos(Psi)*sin(Phi) - cos(Phi)*sin(Psi)*sin(Theta)))/m;
B_out(2,3) = (2*K_t*Omega_3*(cos(Psi)*sin(Phi) - cos(Phi)*sin(Psi)*sin(Theta)))/m;
B_out(2,4) = (2*K_t*Omega_4*(cos(Psi)*sin(Phi) - cos(Phi)*sin(Psi)*sin(Theta)))/m;

B_out(3,1) = -(2*K_t*Omega_1*cos(Phi)*cos(Theta))/m;
B_out(3,2) = -(2*K_t*Omega_2*cos(Phi)*cos(Theta))/m;
B_out(3,3) = -(2*K_t*Omega_3*cos(Phi)*cos(Theta))/m;
B_out(3,4) = -(2*K_t*Omega_4*cos(Phi)*cos(Theta))/m;

B_out(4,1) = -(2*K_t*Omega_1*b)/Ixx;
B_out(4,2) = (2*K_t*Omega_2*b)/Ixx;
B_out(4,3) = (2*K_t*Omega_3*b)/Ixx;
B_out(4,4) = -(2*K_t*Omega_4*b)/Ixx;

B_out(5,1) = (2*K_t*Omega_1*l)/Iyy;
B_out(5,2) = (2*K_t*Omega_2*l)/Iyy;
B_out(5,3) = -(2*K_t*Omega_3*l)/Iyy;
B_out(5,4) = -(2*K_t*Omega_4*l)/Iyy;

B_out(6,1) = (2*K_m*Omega_1)/Izz;
B_out(6,2) = -(2*K_m*Omega_2)/Izz;
B_out(6,3) = (2*K_m*Omega_3)/Izz;
B_out(6,4) = -(2*K_m*Omega_4)/Izz;

end

== matlab function B2_comparison_tool/System 1 - Old/INDI Cascaded/MATLAB Function ==
  data: Ixx input; B_inner output; Iyy input; Izz input; K_m input; K_t input; Omega_1 input; Omega_2 input; Omega_3 input; Omega_4 input; b input; l input
function B_inner = control_allocation_simple_inner(Ixx,Iyy,Izz,K_m,K_t,Omega_1,Omega_2,Omega_3,Omega_4,b,l)

B_inner = zeros(4,4);

B_inner(1,1) = -(2*K_t*Omega_1*b)/Ixx;
B_inner(1,2) = (2*K_t*Omega_2*b)/Ixx;
B_inner(1,3) = (2*K_t*Omega_3*b)/Ixx;
B_inner(1,4) = -(2*K_t*Omega_4*b)/Ixx;

B_inner(2,1) = (2*K_t*Omega_1*l)/Iyy;
B_inner(2,2) = (2*K_t*Omega_2*l)/Iyy;
B_inner(2,3) = -(2*K_t*Omega_3*l)/Iyy;
B_inner(2,4) = -(2*K_t*Omega_4*l)/Iyy;

B_inner(3,1) = (2*K_m*Omega_1)/Izz;
B_inner(3,2) = -(2*K_m*Omega_2)/Izz;
B_inner(3,3) = (2*K_m*Omega_3)/Izz;
B_inner(3,4) = -(2*K_m*Omega_4)/Izz;

B_inner(4,1) = -2*K_t*Omega_1;
B_inner(4,2) = -2*K_t*Omega_2;
B_inner(4,3) = -2*K_t*Omega_3;
B_inner(4,4) = -2*K_t*Omega_4;

end

== matlab function B2_comparison_tool/System 0 - New/INDI Block/MATLAB Function ==
  data: Ixx input; B_out output; Iyy input; Izz input; K_m input; K_t input; Omega_1 input; Omega_2 input; Omega_3 input; Omega_4 input; Phi input; Psi input; Theta input; b input; l input; m input
function B_out = control_allocation_simple(Ixx,Iyy,Izz,K_m,K_t,Omega_1,Omega_2,Omega_3,Omega_4,Phi,Psi,Theta,b,l,m)

B_out = zeros(6,4);

B_out(1,1) = -(2*K_t*Omega_1*(sin(Phi)*sin(Psi) + cos(Phi)*cos(Psi)*sin(Theta)))/m;
B_out(1,2) = -(2*K_t*Omega_2*(sin(Phi)*sin(Psi) + cos(Phi)*cos(Psi)*sin(Theta)))/m;
B_out(1,3) = -(2*K_t*Omega_3*(sin(Phi)*sin(Psi) + cos(Phi)*cos(Psi)*sin(Theta)))/m;
B_out(1,4) = -(2*K_t*Omega_4*(sin(Phi)*sin(Psi) + cos(Phi)*cos(Psi)*sin(Theta)))/m;

B_out(2,1) = (2*K_t*Omega_1*(cos(Psi)*sin(Phi) - cos(Phi)*sin(Psi)*sin(Theta)))/m;
B_out(2,2) = (2*K_t*Omega_2*(cos(Psi)*sin(Phi) - cos(Phi)*sin(Psi)*sin(Theta)))/m;
B_out(2,3) = (2*K_t*Omega_3*(cos(Psi)*sin(Phi) - cos(Phi)*sin(Psi)*sin(Theta)))/m;
B_out(2,4) = (2*K_t*Omega_4*(cos(Psi)*sin(Phi) - cos(Phi)*sin(Psi)*sin(Theta)))/m;

B_out(3,1) = -(2*K_t*Omega_1*cos(Phi)*cos(Theta))/m;
B_out(3,2) = -(2*K_t*Omega_2*cos(Phi)*cos(Theta))/m;
B_out(3,3) = -(2*K_t*Omega_3*cos(Phi)*cos(Theta))/m;
B_out(3,4) = -(2*K_t*Omega_4*cos(Phi)*cos(Theta))/m;

B_out(4,1) = -(2*K_t*Omega_1*b)/Ixx;
B_out(4,2) = (2*K_t*Omega_2*b)/Ixx;
B_out(4,3) = (2*K_t*Omega_3*b)/Ixx;
B_out(4,4) = -(2*K_t*Omega_4*b)/Ixx;

B_out(5,1) = (2*K_t*Omega_1*l)/Iyy;
B_out(5,2) = (2*K_t*Omega_2*l)/Iyy;
B_out(5,3) = -(2*K_t*Omega_3*l)/Iyy;
B_out(5,4) = -(2*K_t*Omega_4*l)/Iyy;

B_out(6,1) = (2*K_m*Omega_1)/Izz;
B_out(6,2) = -(2*K_m*Omega_2)/Izz;
B_out(6,3) = (2*K_m*Omega_3)/Izz;
B_out(6,4) = -(2*K_m*Omega_4)/Izz;

end

== matlab function B2_comparison_tool/System 1 - Old/INDI Cascaded/MATLAB Function1 ==
  data: T input; B_outer output; Phi input; Theta input; Psi input; m input
function B_outer = control_allocation_simple_outer(T,Phi,Theta,Psi,m)

B_outer = zeros(3,3);

B_outer(1,1) = (T*(cos(Phi)*sin(Psi) - cos(Psi)*sin(Phi)*sin(Theta)))/m;  
B_outer(1,2) = (T*cos(Phi)*cos(Psi)*cos(Theta))/m;
B_outer(1,3) = (sin(Phi)*sin(Psi) + cos(Phi)*cos(Psi)*sin(Theta))/m;

B_outer(2,1) = -(T*(cos(Phi)*cos(Psi) + sin(Phi)*sin(Psi)*sin(Theta)))/m;
B_outer(2,2) = (T*cos(Phi)*cos(Theta)*sin(Psi))/m;
B_outer(2,3) = -(cos(Psi)*sin(Phi) - cos(Phi)*sin(Psi)*sin(Theta))/m;

B_outer(3,1) = -(T*cos(Theta)*sin(Phi))/m;                         
B_outer(3,2) = -(T*cos(Phi)*sin(Theta))/m;
B_outer(3,3) = (cos(Phi)*cos(Theta))/m; 

end

== matlab function B2_comparison_tool/System 1 - Old/INDI Cascaded w// Actuator Consideration/MATLAB Function ==
  data: Ixx input; B_inner output; Iyy input; Izz input; K_m input; K_t input; Omega_1 input; Omega_2 input; Omega_3 input; Omega_4 input; b input; l input; K_act_inner input
function B_inner = control_allocation_simple_inner(Ixx,Iyy,Izz,K_m,K_t,Omega_1,Omega_2,Omega_3,Omega_4,b,l,K_act_inner)

B_inner = zeros(4,4);

B_inner(1,1) = -(2*K_t*Omega_1*b)/Ixx;
B_inner(1,2) = (2*K_t*Omega_2*b)/Ixx;
B_inner(1,3) = (2*K_t*Omega_3*b)/Ixx;
B_inner(1,4) = -(2*K_t*Omega_4*b)/Ixx;

B_inner(2,1) = (2*K_t*Omega_1*l)/Iyy;
B_inner(2,2) = (2*K_t*Omega_2*l)/Iyy;
B_inner(2,3) = -(2*K_t*Omega_3*l)/Iyy;
B_inner(2,4) = -(2*K_t*Omega_4*l)/Iyy;

B_inner(3,1) = (2*K_m*Omega_1)/Izz;
B_inner(3,2) = -(2*K_m*Omega_2)/Izz;
B_inner(3,3) = (2*K_m*Omega_3)/Izz;
B_inner(3,4) = -(2*K_m*Omega_4)/Izz;

B_inner(4,1) = -2*K_t*Omega_1;
B_inner(4,2) = -2*K_t*Omega_2;
B_inner(4,3) = -2*K_t*Omega_3;
B_inner(4,4) = -2*K_t*Omega_4;

% actuator compensation
B_inner = K_act_inner*B_inner;

end

== matlab function B2_comparison_tool/System 1 - Old/INDI Cascaded w// Actuator Consideration/MATLAB Function1 ==
  data: T input; B_outer output; Phi input; Theta input; Psi input; m input
function B_outer = control_allocation_simple_outer(T,Phi,Theta,Psi,m)

B_outer = zeros(3,3);

B_outer(1,1) = (T*(cos(Phi)*sin(Psi) - cos(Psi)*sin(Phi)*sin(Theta)))/m;  
B_outer(1,2) = (T*cos(Phi)*cos(Psi)*cos(Theta))/m;
B_outer(1,3) = (sin(Phi)*sin(Psi) + cos(Phi)*cos(Psi)*sin(Theta))/m;

B_outer(2,1) = -(T*(cos(Phi)*cos(Psi) + sin(Phi)*sin(Psi)*sin(Theta)))/m;
B_outer(2,2) = (T*cos(Phi)*cos(Theta)*sin(Psi))/m;
B_outer(2,3) = -(cos(Psi)*sin(Phi) - cos(Phi)*sin(Psi)*sin(Theta))/m;

B_outer(3,1) = -(T*cos(Theta)*sin(Phi))/m;                         
B_outer(3,2) = -(T*cos(Phi)*sin(Theta))/m;
B_outer(3,3) = (cos(Phi)*cos(Theta))/m; 

end

== matlab function B2_comparison_tool/System 1 - Old/INDI Cascaded w// PD controller/MATLAB Function ==
  data: Ixx input; B_inner output; Iyy input; Izz input; K_m input; K_t input; Omega_1 input; Omega_2 input; Omega_3 input; Omega_4 input; b input; l input
function B_inner = control_allocation_simple_inner(Ixx,Iyy,Izz,K_m,K_t,Omega_1,Omega_2,Omega_3,Omega_4,b,l)

B_inner = zeros(4,4);

B_inner(1,1) = -(2*K_t*Omega_1*b)/Ixx;
B_inner(1,2) = (2*K_t*Omega_2*b)/Ixx;
B_inner(1,3) = (2*K_t*Omega_3*b)/Ixx;
B_inner(1,4) = -(2*K_t*Omega_4*b)/Ixx;

B_inner(2,1) = (2*K_t*Omega_1*l)/Iyy;
B_inner(2,2) = (2*K_t*Omega_2*l)/Iyy;
B_inner(2,3) = -(2*K_t*Omega_3*l)/Iyy;
B_inner(2,4) = -(2*K_t*Omega_4*l)/Iyy;

B_inner(3,1) = (2*K_m*Omega_1)/Izz;
B_inner(3,2) = -(2*K_m*Omega_2)/Izz;
B_inner(3,3) = (2*K_m*Omega_3)/Izz;
B_inner(3,4) = -(2*K_m*Omega_4)/Izz;

B_inner(4,1) = -2*K_t*Omega_1;
B_inner(4,2) = -2*K_t*Omega_2;
B_inner(4,3) = -2*K_t*Omega_3;
B_inner(4,4) = -2*K_t*Omega_4;

end

== matlab function B2_comparison_tool/System 1 - Old/INDI Cascaded w// PD controller/MATLAB Function1 ==
  data: T input; B_outer output; Phi input; Theta input; Psi input; m input
function B_outer = control_allocation_simple_outer(T,Phi,Theta,Psi,m)

B_outer = zeros(3,3);

B_outer(1,1) = (T*(cos(Phi)*sin(Psi) - cos(Psi)*sin(Phi)*sin(Theta)))/m;  
B_outer(1,2) = (T*cos(Phi)*cos(Psi)*cos(Theta))/m;
B_outer(1,3) = (sin(Phi)*sin(Psi) + cos(Phi)*cos(Psi)*sin(Theta))/m;

B_outer(2,1) = -(T*(cos(Phi)*cos(Psi) + sin(Phi)*sin(Psi)*sin(Theta)))/m;
B_outer(2,2) = (T*cos(Phi)*cos(Theta)*sin(Psi))/m;
B_outer(2,3) = -(cos(Psi)*sin(Phi) - cos(Phi)*sin(Psi)*sin(Theta))/m;

B_outer(3,1) = -(T*cos(Theta)*sin(Phi))/m;                         
B_outer(3,2) = -(T*cos(Phi)*sin(Theta))/m;
B_outer(3,3) = (cos(Phi)*cos(Theta))/m; 

end

== matlab function B2_comparison_tool/System 1 - Old/INDI w// RSPI/MATLAB Function ==
  data: Ixx input; u_out output; Iyy input; Izz input; K_m input; K_t input; Omega_1 input; Omega_2 input; Omega_3 input; Omega_4 input; Phi input; Psi input; Theta input; b input; l input; m input; dv input; desired_u input; max_omega_motor input; max_motor_rate input; sampling_time input; max_iter input
function u_out = control_allocation_simple(Ixx,Iyy,Izz,K_m,K_t,Omega_1,Omega_2,Omega_3,Omega_4,Phi,Psi,Theta,b,l,m,dv,desired_u,max_omega_motor,max_motor_rate,sampling_time,max_iter)

%% Identify and evaluate effectiveness matrix

B_out = zeros(6,4);

B_out(1,1) = -(2*K_t*Omega_1*(sin(Phi)*sin(Psi) + cos(Phi)*cos(Psi)*sin(Theta)))/m;
B_out(1,2) = -(2*K_t*Omega_2*(sin(Phi)*sin(Psi) + cos(Phi)*cos(Psi)*sin(Theta)))/m;
B_out(1,3) = -(2*K_t*Omega_3*(sin(Phi)*sin(Psi) + cos(Phi)*cos(Psi)*sin(Theta)))/m;
B_out(1,4) = -(2*K_t*Omega_4*(sin(Phi)*sin(Psi) + cos(Phi)*cos(Psi)*sin(Theta)))/m;

B_out(2,1) = (2*K_t*Omega_1*(cos(Psi)*sin(Phi) - cos(Phi)*sin(Psi)*sin(Theta)))/m;
B_out(2,2) = (2*K_t*Omega_2*(cos(Psi)*sin(Phi) - cos(Phi)*sin(Psi)*sin(Theta)))/m;
B_out(2,3) = (2*K_t*Omega_3*(cos(Psi)*sin(Phi) - cos(Phi)*sin(Psi)*sin(Theta)))/m;
B_out(2,4) = (2*K_t*Omega_4*(cos(Psi)*sin(Phi) - cos(Phi)*sin(Psi)*sin(Theta)))/m;

B_out(3,1) = -(2*K_t*Omega_1*cos(Phi)*cos(Theta))/m;
B_out(3,2) = -(2*K_t*Omega_2*cos(Phi)*cos(Theta))/m;
B_out(3,3) = -(2*K_t*Omega_3*cos(Phi)*cos(Theta))/m;
B_out(3,4) = -(2*K_t*Omega_4*cos(Phi)*cos(Theta))/m;

B_out(4,1) = -(2*K_t*Omega_1*b)/Ixx;
B_out(4,2) = (2*K_t*Omega_2*b)/Ixx;
B_out(4,3) = (2*K_t*Omega_3*b)/Ixx;
B_out(4,4) = -(2*K_t*Omega_4*b)/Ixx;

B_out(5,1) = (2*K_t*Omega_1*l)/Iyy;
B_out(5,2) = (2*K_t*Omega_2*l)/Iyy;
B_out(5,3) = -(2*K_t*Omega_3*l)/Iyy;
B_out(5,4) = -(2*K_t*Omega_4*l)/Iyy;

B_out(6,1) = (2*K_m*Omega_1)/Izz;
B_out(6,2) = -(2*K_m*Omega_2)/Izz;
B_out(6,3) = (2*K_m*Omega_3)/Izz;
B_out(6,4) = -(2*K_m*Omega_4)/Izz;

% get current u
actual_u = [Omega_1, Omega_2, Omega_3, Omega_4];

% modify pseudo control to mimimize u
dv = dv + B_out * (actual_u' - desired_u);

%% Apply gains to normalize the effectiveness matrix

gain_motor = max_omega_motor/2;
B_out = B_out * gain_motor;

%% Apply RSPI

% build max e min u array
u_max = [max_omega_motor, max_omega_motor, max_omega_motor, max_omega_motor];
u_min = [0,0,0,0];

% get maximum rate
du_rate_max = zeros(1,length(u_max));
du_rate_max(1:4) = max_motor_rate*sampling_time;
du_rate_min = - du_rate_max;

max_du = zeros(1,length(u_max));
min_du = zeros(1,length(u_max));
%Compute the maximum and minimum control input available for each channel: 
for i=1:length(u_max)
    max_du(i) = min( u_max(i) , actual_u(i) + du_rate_max(i));
    min_du(i) = max( u_min(i) , actual_u(i) + du_rate_min(i));
end

max_du =  u_max;
min_du =  u_min;

max_du_scaled = max_du;
min_du_scaled = min_du;
max_du_scaled = max_du_scaled / gain_motor;
min_du_scaled = min_du_scaled / gain_motor;

max_du_scaled = max_du_scaled';
min_du_scaled = min_du_scaled';

sensibility_pseudo_control = 0.001;

% Multiply the pseudo control with the inversion of the control effectiveness to get the control inputs 
B_inv = pinv(B_out);
du_scaled = B_inv * dv; 

B_new = B_out;

locked_actuator = zeros(1,length(u_max));
Scaling_array = ones(1,length(u_max));
reached_pseudo_control = 0;

%Build the scaling array and check for actuator saturation, if so modify the B matrix: 
for i=1:length(u_max)
    if(du_scaled(i) > 0 && locked_actuator(i) == 0)
        Scaling_array(i) = min( 1 , max_du_scaled(i) / du_scaled(i) );        
    elseif(du_scaled(i) < 0 && locked_actuator(i) == 0 )
        Scaling_array(i) = min( 1 , min_du_scaled(i) / du_scaled(i) );
    end     
end

%If we have saturation reduce the control input and prepare for the next iteration 
if( sum(Scaling_array) < length(Scaling_array) )
    %Determine saturated actuators
    locked_actuator( abs(Scaling_array - min(Scaling_array)) < 0.001 ) = 1;
    %Zeroing the column of the effectiveness matrix related to saturated actuators
    B_new(:, locked_actuator == 1 ) = 0;
    %Scale the control input array: 
    du_scaled_s = du_scaled.*min(Scaling_array);
    %Compute the new maximum achievable pseudo control increment associated to the new control input: 
    du_scaled_tot = du_scaled_s;
    dv_ach = B_out * du_scaled_s;

    %Compute the new objective for the pseudo control of the next iteration 
    new_dv = dv - dv_ach;

    %Check if we satisfy the pseudo control with this actuator configuration: 
    if( sum(abs(new_dv)) < sensibility_pseudo_control ) 
        reached_pseudo_control = 1;
    end  

%If we don't saturate just return the actuator increment and that's it    
else
    du_scaled_tot = du_scaled;
    new_dv = dv;
    du_scaled_s = du_scaled.*min(Scaling_array);
end


%Begin the iterative process if we are saturating one of the actuators
j = 1;
while( sum(Scaling_array) < length(Scaling_array) && j <= max_iter && reached_pseudo_control == 0)
    
    %Compute the new control input with the modified B matrix 
    B_new_inv = pinv(B_new);
    du_scaled = B_new_inv * new_dv; 

    %Build the maximum and minimum delta u available for each channel: 
    max_du_scaled = max_du_scaled - du_scaled_s;
    min_du_scaled = min_du_scaled - du_scaled_s;
    
    Scaling_array = ones(1,length(u_max));
    %Build the scaling array and check for actuator saturation, if so modify the B matrix: 
    for i=1:length(u_max)
        if(du_scaled(i) > 0 && locked_actuator(i) == 0)
            Scaling_array(i) = min( 1 , max_du_scaled(i) / du_scaled(i) );        
        elseif(du_scaled(i) < 0 && locked_actuator(i) == 0 )
            Scaling_array(i) = min( 1 , min_du_scaled(i) / du_scaled(i) );
        end     
    end

    %If we have saturation reduce the control input and prepare for the next iteration 
    if(sum(Scaling_array) < length(Scaling_array))
        %Determine saturated actuators
        locked_actuator( abs( Scaling_array - min(Scaling_array)) < 0.01 ) = 1;
        B_new(:, abs( Scaling_array - min(Scaling_array)) < 0.01 ) = 0;
        %Scale the control input array: 
        du_scaled_s = du_scaled.*min(Scaling_array);
        %Compute the new maximum achievable pseudo control increment associated to the new control input: 
        du_scaled_tot = du_scaled_tot + du_scaled_s;
        dv_ach = B_out * du_scaled_s;   

        %Compute the new objective for the pseudo control of the next iteration 
        new_dv = new_dv - dv_ach;

        %Check if we satisfy the pseudo control with this actuator configuration: 
        if( sum(abs(new_dv)) < sensibility_pseudo_control ) 
            reached_pseudo_control = 1;
        end  

    %If we don't saturate just return the actuator increment and that's it    
    else
        du_scaled_tot = du_scaled_tot + du_scaled;
    end    
   
    %Increase the counter: 
    j = j + 1;
    
end

du = du_scaled_tot;
%Scale back the increment to remove the normalization
du = du * gain_motor;

u_out =  du' + desired_u';

end

== matlab function B2_comparison_tool/System 0 - New/INDI Cascaded w// State Compensation on qdd/MATLAB Function1 ==
  data: T input; B_outer output; Phi input; Theta input; Psi input; m input
function B_outer = control_allocation_simple_outer(T,Phi,Theta,Psi,m)

B_outer = zeros(3,3);

B_outer(1,1) = (T*(cos(Phi)*sin(Psi) - cos(Psi)*sin(Phi)*sin(Theta)))/m;  
B_outer(1,2) = (T*cos(Phi)*cos(Psi)*cos(Theta))/m;
B_outer(1,3) = (sin(Phi)*sin(Psi) + cos(Phi)*cos(Psi)*sin(Theta))/m;

B_outer(2,1) = -(T*(cos(Phi)*cos(Psi) + sin(Phi)*sin(Psi)*sin(Theta)))/m;
B_outer(2,2) = (T*cos(Phi)*cos(Theta)*sin(Psi))/m;
B_outer(2,3) = -(cos(Psi)*sin(Phi) - cos(Phi)*sin(Psi)*sin(Theta))/m;

B_outer(3,1) = -(T*cos(Theta)*sin(Phi))/m;                         
B_outer(3,2) = -(T*cos(Phi)*sin(Theta))/m;
B_outer(3,3) = (cos(Phi)*cos(Theta))/m; 

end

== matlab function B2_comparison_tool/System 0 - New/INDI Cascaded w// State Compensation on qdd/STATE COMPENSATION BLOCK/Mathematical Derivation ==
  data: r_plate input; qdd_x output; l_plate input; Iyy input; rho input; u_b input; v_b input; w_b input; alpha input; ud_b input; vd_b input; wd_b input; alphad input
function qdd_x = fcn(r_plate, l_plate, Iyy, rho, u_b, v_b, w_b, alpha, ud_b, vd_b, wd_b, alphad)

S_plate = pi*r_plate^2;

qdd_x = (S_plate*l_plate*rho*(cos(alpha)*((33*alpha)/10000 + 997/1000) ...
    + sin(alpha)*((57*alpha)/2500 + 21/500))*(2*u_b*ud_b + 2*v_b*vd_b + 2*w_b*wd_b))/(2*Iyy) ...
    + (S_plate*l_plate*rho*(u_b^2 + v_b^2 + w_b^2)*((33*alphad*cos(alpha))/10000 ...
    + (57*alphad*sin(alpha))/2500 + alphad*cos(alpha)*((57*alpha)/2500 + 21/500) ...
    - alphad*sin(alpha)*((33*alpha)/10000 + 997/1000)))/(2*Iyy);

end
